simulink model "test_RS_flipflop_statemachine"  (R2021a)
settings: Solver=FixedStepDiscrete  StartTime=0.0  StopTime=210*10e-8  RelTol=1e-3
values from neighbouring files (symbols this model uses):
  t_ADC = 1/f_ADC    (= 1e-05)    [uz_6ph_pu_vsd_voltages_init.m]    (also in uz_mpc_6ph_init.m; uz_mpc_6ph_state_machine_init.m; uz_typeconv_init.m)
  t_clock = 1/f_clock    (= 1e-08)    [uz_6ph_pu_vsd_voltages_init.m]    (also in uz_mpc_6ph_init.m; uz_mpc_6ph_state_machine_init.m; uz_typeconv_init.m)
libraries: simulink x15, simulink_extras x1
settings Model: DataTypeOverride=Off  Creator=micha  LastModifiedBy=micha
settings SolverCC: AlgebraicLoopSolver=TrustRegion
settings DataIOCC: LimitDataPoints=on  SaveOutput=off  SaveTime=off
settings OptimizationCC: BlockReduction=off  ConditionallyExecuteInputs=off  DefaultParameterBehavior=Inlined  LifeSpan=inf
settings DebuggingCC: AlgebraicLoopMsg=error  SingleTaskRateTransMsg=error  AllowSymbolicDim=off  StrictBusMsg=ErrorOnBusTreatedAsVector  SFUnexpectedBacktrackingDiag=warning  SFNoUnconditionalDefaultTransitionDiag=warning  SFExecutionAtInitializationDiag=none  SFMachineParentedDataDiag=warning  ArithmeticOperatorsInVariantConditions=warning
settings HardwareCC: ProdBitPerPointer=32  ProdBitPerSizeT=32  ProdBitPerPtrDiffT=32  ProdLargestAtomicFloat=None  ProdIntDivRoundTo=Undefined  ProdEndianess=Unspecified  ProdWordSize=32  ProdHWDeviceType=ASIC/FPGA->ASIC/FPGA  ProdEqTarget=off
settings SFSimCC: SimUseLocalCustomCode=off  CustomCodeUndefinedFunction=UseInterfaceOnly
settings RTWCC: RTWUseLocalCustomCode=off
settings CodeAppCC: StateflowObjectComments=on
settings GRTTargetCC: TargetLangStandard=C89/C90 (ANSI)
settings ConfigComp: CovScope=ReferencedModels  CovMetricSettings=dw  CovSaveCumulativeToWorkspaceVar=on  CovSaveSingleToWorkspaceVar=on  CovExternalEMLEnable=off  CovSFcnEnable=off

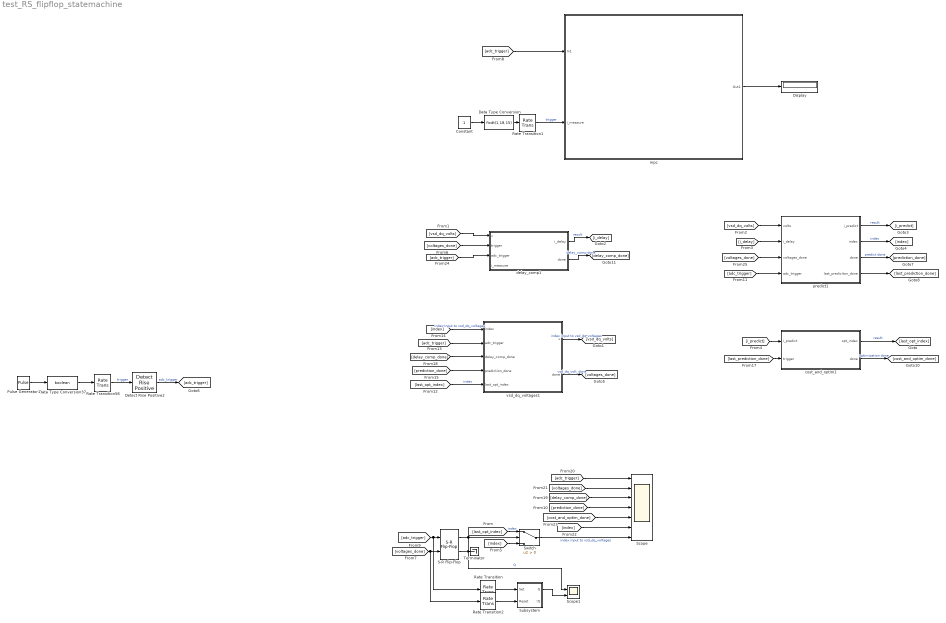
== system test_RS_flipflop_statemachine ==
  Constant : Constant
  Data Type Conversion : DataTypeConversion  OutDataTypeStr=fixdt(1,18,15)
  Data Type Conversion37 : DataTypeConversion  OutDataTypeStr=boolean
  Detect Rise Positive2 : simulink/Logic and Bit Operations/Detect Rise Positive  vinit=0  OutDataTypeStr=boolean
  Display : Display
  Pulse Generator1 : DiscretePulseGenerator  PulseType=Time based  Period=t_ADC  PulseWidth=5
  Rate Transition{,1..2,58} (4 alike) : RateTransition  OutPortSampleTime=t_clock
  S-R Flip-Flop : simulink_extras/Flip Flops/S-R Flip-Flop  initial_condition=0
  Scope : Scope  NumInputPorts=7
  Scope1 : Scope  NumInputPorts=2
  Subsystem : Subsystem
  Switch : Switch  Criteria=u2 > Threshold
  Terminator : Terminator
  cost_and_optim1 : Subsystem
  delay_comp1 : Subsystem
  mpc : Subsystem  TreatAsAtomicUnit=on
  predict1 : Subsystem
  vsd_dq_voltages1 : Subsystem
  wires:
  Data Type Conversion37/1 -> Rate Transition58/1
  Rate Transition58/1 -> Detect Rise Positive2/1  "trigger"
  Pulse Generator1/1 -> Data Type Conversion37/1
  S-R Flip-Flop/1 -> Scope1/1, Switch/2  "Q"
  [last_opt_index] -> Switch/1  "index"
  [index] -> vsd_dq_voltages1/1(index)  "index input to vsd_dq_voltages"
  S-R Flip-Flop/2 -> Terminator/1
  Detect Rise Positive2/1 -> [adc_trigger]  "adc_trigger"
  vsd_dq_voltages1/2(done) -> [voltages_done]  "vsd_dq_volt_done"
  predict1/3(done) -> [prediction_done]  "predict done"
  predict1/2(index) -> [index]  "index"
  cost_and_optim1/1(opt_index) -> [last_opt_index]  "result"
  [vsd_dq_volts] -> delay_comp1/1(v)
  [vsd_dq_volts] -> predict1/1(volts)
  delay_comp1/1(i_delay) -> [i_delay]  "result"
  [i_delay] -> predict1/2(i_delay)
  predict1/1(i_predict) -> [i_predict]  "result"
  [i_predict] -> cost_and_optim1/1(i_predict)
  [index] -> Switch/3
  [voltages_done] -> delay_comp1/2(trigger)
  [voltages_done] -> Rate Transition2/1, S-R Flip-Flop/2
  [adc_trigger] -> Rate Transition/1, S-R Flip-Flop/1
  [adc_trigger] -> predict1/4(adc_trigger)
  [last_opt_index] -> vsd_dq_voltages1/5(last_opt_index)  "index"
  [adc_trigger] -> vsd_dq_voltages1/2(adc_trigger)
  vsd_dq_voltages1/1(v) -> [vsd_dq_volts]  "index input to vsd_dq_voltages"
  [prediction_done] -> vsd_dq_voltages1/4(prediction_done)
  [last_prediction_done] -> cost_and_optim1/2(trigger)
  [delay_comp_done] -> vsd_dq_voltages1/3(delay_comp_done)
  Switch/1 -> Scope/7  "index input to vsd_dq_voltages"
  [delay_comp_done] -> Scope/3
  [adc_trigger] -> Scope/1
  [voltages_done] -> Scope/2
  [index] -> Scope/6
  cost_and_optim1/2(done) -> [cost_and_optim_done]  "optimization done"
  [cost_and_optim_done] -> Scope/5
  [adc_trigger] -> delay_comp1/3(adc_trigger)
  delay_comp1/2(done) -> [delay_comp_done]  "delay_comp done"
  [voltages_done] -> predict1/3(voltages_done)
  predict1/4(last_prediciton_done) -> [last_prediction_done]
  [prediction_done] -> Scope/4
  [adc_trigger] -> mpc/1(In1)
  Rate Transition1/1 -> mpc/2(i_measure)  "trigger"
  Constant/1 -> Data Type Conversion/1
  Data Type Conversion/1 -> Rate Transition1/1
  mpc/1(Out1) -> Display/1
  Subsystem/1(Q) -> Scope1/2
  Rate Transition/1 -> Subsystem/1(Set)
  Rate Transition2/1 -> Subsystem/2(Reset)

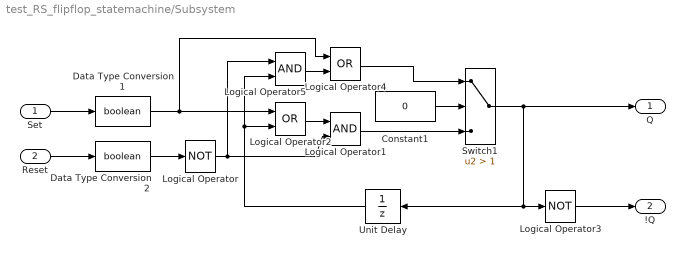
== system test_RS_flipflop_statemachine/Subsystem ==
  Set : Inport
  Reset : Inport  Port=2
  Constant1 : Constant  Value=0  SampleTime=-1
  Data Type Conversion1 : DataTypeConversion  OutDataTypeStr=boolean
  Data Type Conversion2 : DataTypeConversion  OutDataTypeStr=boolean
  Logical Operator : Logic  Operator=NOT  AllPortsSameDT=off  OutDataTypeStr=boolean
  Logical Operator1 : Logic  AllPortsSameDT=off  OutDataTypeStr=boolean
  Logical Operator2 : Logic  Operator=OR  AllPortsSameDT=off  OutDataTypeStr=boolean
  Logical Operator3 : Logic  Operator=NOT  AllPortsSameDT=off  OutDataTypeStr=boolean
  Logical Operator4 : Logic  Operator=OR  AllPortsSameDT=off  OutDataTypeStr=boolean
  Logical Operator5 : Logic  AllPortsSameDT=off  OutDataTypeStr=boolean
  Switch1 : Switch  Criteria=u2 > Threshold  Threshold=1
  Unit Delay : UnitDelay  SampleTime=t_clock  HasFrameUpgradeWarning=on
  Q : Outport  VectorParamsAs1DForOutWhenUnconnected=off
  !Q : Outport  Port=2  VectorParamsAs1DForOutWhenUnconnected=off
  wires:
  Logical Operator/1 -> Logical Operator1/2, Logical Operator5/1
  Reset/1 -> Data Type Conversion2/1
  Constant1/1 -> Switch1/2
  Logical Operator4/1 -> Switch1/1
  Data Type Conversion1/1 -> Logical Operator2/1, Logical Operator4/1
  Switch1/1 -> Q/1, Unit Delay/1, Logical Operator3/1
  Logical Operator3/1 -> !Q/1
  Set/1 -> Data Type Conversion1/1
  Logical Operator2/1 -> Logical Operator1/1
  Unit Delay/1 -> Logical Operator2/2, Logical Operator5/2
  Logical Operator5/1 -> Logical Operator4/2
  Logical Operator1/1 -> Switch1/3
  Data Type Conversion2/1 -> Logical Operator/1

== system test_RS_flipflop_statemachine/cost_and_optim1 ==
  i_predict : Inport
  trigger : Inport  Port=2
  Add : Sum
  Constant : Constant  Value=42  OutDataTypeStr=uint32  SampleTime=-1
  Delay{,1..4} (5 alike) : Delay  DelayLength=1
  Detect Rise Positive : simulink/Logic and Bit Operations/Detect Rise Positive  vinit=0  OutDataTypeStr=boolean
  Switch : Switch  Criteria=u2 > Threshold
  Terminator : Terminator
  opt_index : Outport  VectorParamsAs1DForOutWhenUnconnected=off
  done : Outport  Port=2  VectorParamsAs1DForOutWhenUnconnected=off
  wires:
  trigger/1 -> Delay/1
  Delay/1 -> Detect Rise Positive/1
  Delay1/1 -> done/1
  Detect Rise Positive/1 -> Delay1/1, Switch/2
  Delay2/1 -> Switch/3
  Switch/1 -> Add/1, Add/2, Delay2/1
  i_predict/1 -> Delay3/1
  Delay3/1 -> Switch/1
  Delay4/1 -> opt_index/1
  Constant/1 -> Delay4/1
  Add/1 -> Terminator/1

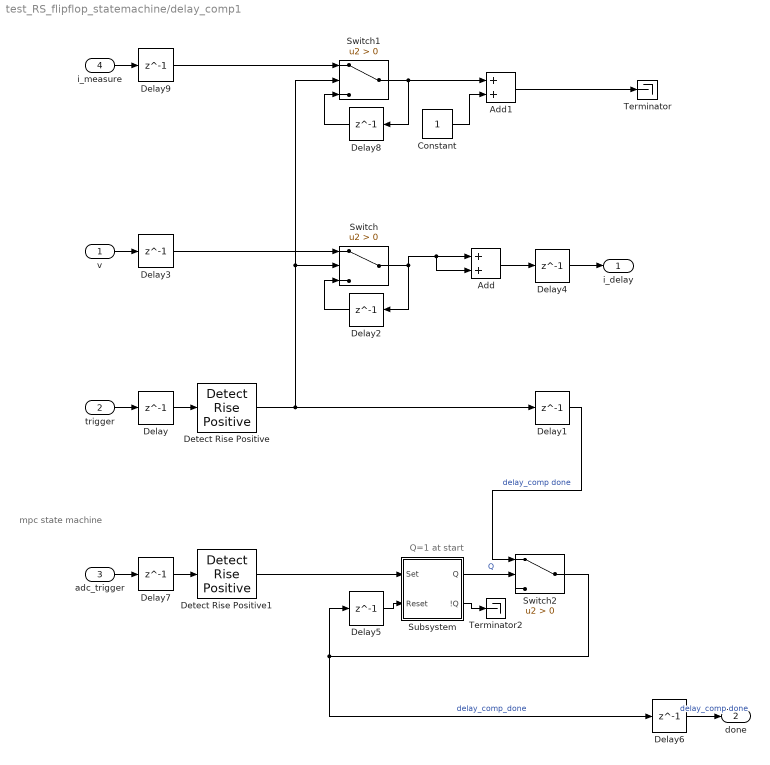
== system test_RS_flipflop_statemachine/delay_comp1 ==
  note: mpc state machine
  note: Q=1 at start
  v : Inport
  trigger : Inport  Port=2
  adc_trigger : Inport  Port=3
  i_measure : Inport  Port=4
  Add : Sum
  Add1 : Sum  AccumDataTypeStr=fixdt(1,18,15)
  Constant : Constant  OutDataTypeStr=fixdt(1,27,24)  SampleTime=-1
  Delay{,1..9} (10 alike) : Delay  DelayLength=1
  Detect Rise Positive : simulink/Logic and Bit Operations/Detect Rise Positive  vinit=0  OutDataTypeStr=boolean
  Detect Rise Positive1 : simulink/Logic and Bit Operations/Detect Rise Positive  vinit=0  OutDataTypeStr=boolean
  Subsystem : Subsystem
  Switch : Switch  Criteria=u2 > Threshold
  Switch1 : Switch  Criteria=u2 > Threshold
  Switch2 : Switch  Criteria=u2 > Threshold
  Terminator : Terminator
  Terminator2 : Terminator
  i_delay : Outport  VectorParamsAs1DForOutWhenUnconnected=off
  done : Outport  Port=2  VectorParamsAs1DForOutWhenUnconnected=off
  wires:
  trigger/1 -> Delay/1
  Delay/1 -> Detect Rise Positive/1
  Delay2/1 -> Switch/3
  Switch/1 -> Add/2, Add/1, Delay2/1
  v/1 -> Delay3/1
  Delay3/1 -> Switch/1
  Delay4/1 -> i_delay/1
  Add/1 -> Delay4/1
  Switch2/1 -> Delay5/1, Delay6/1  "delay_comp_done"
  Subsystem/1(Q) -> Switch2/2  "Q"
  Delay7/1 -> Detect Rise Positive1/1
  Subsystem/2(!Q) -> Terminator2/1
  Delay5/1 -> Subsystem/2(Reset)
  Delay1/1 -> Switch2/1  "delay_comp done"
  Delay6/1 -> done/1  "delay_comp done"
  adc_trigger/1 -> Delay7/1
  Detect Rise Positive1/1 -> Subsystem/1(Set)
  Detect Rise Positive/1 -> Delay1/1, Switch1/2, Switch/2
  i_measure/1 -> Delay9/1
  Switch1/1 -> Add1/1, Delay8/1
  Delay8/1 -> Switch1/3
  Delay9/1 -> Switch1/1
  Constant/1 -> Add1/2
  Add1/1 -> Terminator/1

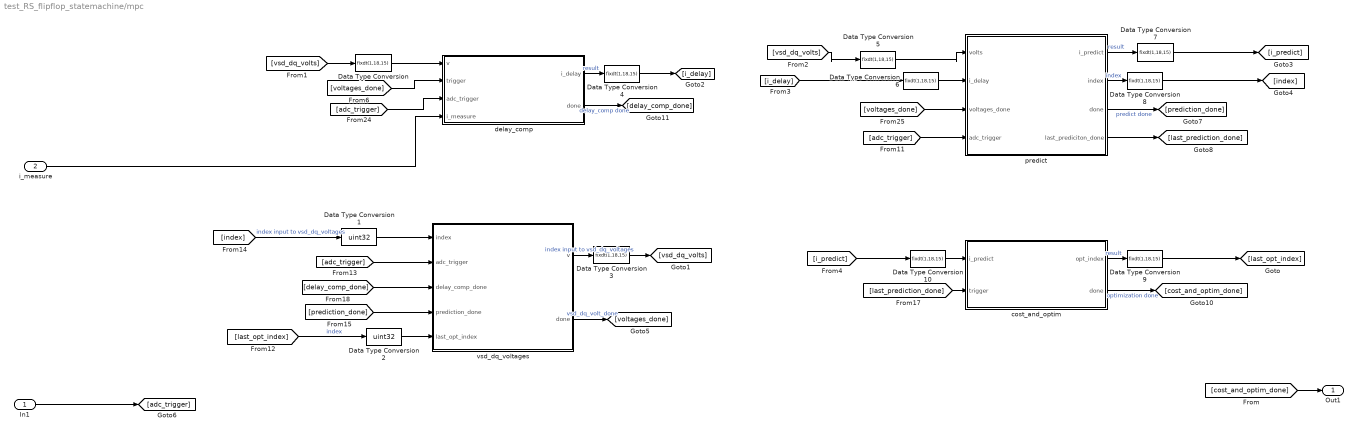
== system test_RS_flipflop_statemachine/mpc ==
  In1 : Inport
  i_measure : Inport  Port=2
  Data Type Conversion{,3..10} (9 alike) : DataTypeConversion  OutDataTypeStr=fixdt(1,18,15)
  Data Type Conversion1 : DataTypeConversion  OutDataTypeStr=uint32
  Data Type Conversion2 : DataTypeConversion  OutDataTypeStr=uint32
  cost_and_optim : Subsystem
  delay_comp : Subsystem
  predict : Subsystem
  vsd_dq_voltages : Subsystem
  Out1 : Outport
  wires:
  cost_and_optim/2(done) -> [cost_and_optim_done]  "optimization done"
  [voltages_done] -> predict/3(voltages_done)
  predict/4(last_prediciton_done) -> [last_prediction_done]
  [prediction_done] -> vsd_dq_voltages/4(prediction_done)
  delay_comp/2(done) -> [delay_comp_done]  "delay_comp done"
  [adc_trigger] -> vsd_dq_voltages/2(adc_trigger)
  [adc_trigger] -> predict/4(adc_trigger)
  [voltages_done] -> delay_comp/2(trigger)
  [vsd_dq_volts] -> Data Type Conversion/1
  [vsd_dq_volts] -> Data Type Conversion5/1
  [last_opt_index] -> Data Type Conversion2/1  "index"
  [i_delay] -> Data Type Conversion6/1
  delay_comp/1(i_delay) -> Data Type Conversion4/1  "result"
  cost_and_optim/1(opt_index) -> Data Type Conversion9/1  "result"
  vsd_dq_voltages/1(v) -> Data Type Conversion3/1  "index input to vsd_dq_voltages"
  [i_predict] -> Data Type Conversion10/1
  predict/1(i_predict) -> Data Type Conversion7/1  "result"
  [last_prediction_done] -> cost_and_optim/2(trigger)
  [index] -> Data Type Conversion1/1  "index input to vsd_dq_voltages"
  predict/3(done) -> [prediction_done]  "predict done"
  vsd_dq_voltages/2(done) -> [voltages_done]  "vsd_dq_volt_done"
  predict/2(index) -> Data Type Conversion8/1  "index"
  [delay_comp_done] -> vsd_dq_voltages/3(delay_comp_done)
  [adc_trigger] -> delay_comp/3(adc_trigger)
  In1/1 -> [adc_trigger]
  [cost_and_optim_done] -> Out1/1
  i_measure/1 -> delay_comp/4(i_measure)
  Data Type Conversion/1 -> delay_comp/1(v)
  Data Type Conversion1/1 -> vsd_dq_voltages/1(index)
  Data Type Conversion2/1 -> vsd_dq_voltages/5(last_opt_index)
  Data Type Conversion3/1 -> [vsd_dq_volts]
  Data Type Conversion4/1 -> [i_delay]
  Data Type Conversion5/1 -> predict/1(volts)
  Data Type Conversion6/1 -> predict/2(i_delay)
  Data Type Conversion7/1 -> [i_predict]
  Data Type Conversion8/1 -> [index]
  Data Type Conversion9/1 -> [last_opt_index]
  Data Type Conversion10/1 -> cost_and_optim/1(i_predict)

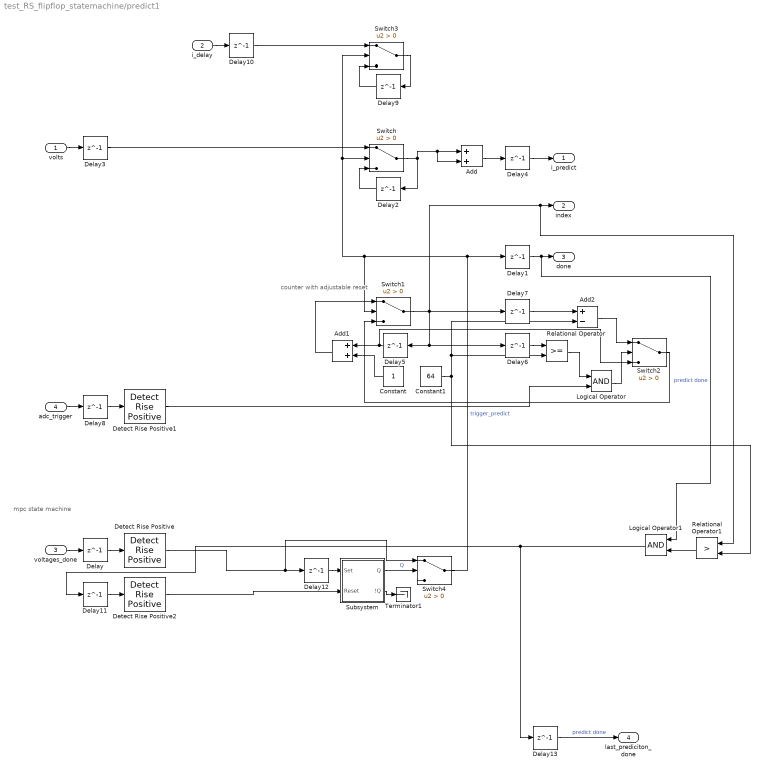
== system test_RS_flipflop_statemachine/predict1 ==
  note: counter with adjustable reset
  note: mpc state machine
  volts : Inport
  i_delay : Inport  Port=2
  voltages_done : Inport  Port=3
  adc_trigger : Inport  Port=4
  Add : Sum
  Add1 : Sum  AccumDataTypeStr=uint32
  Add2 : Sum  Inputs=+-  AccumDataTypeStr=uint32
  Constant : Constant  OutDataTypeStr=uint32  SampleTime=-1
  Constant1 : Constant  Value=64  OutDataTypeStr=uint32  SampleTime=-1
  Delay{,1..4,8..13} (11 alike) : Delay  DelayLength=1
  Delay5 : Delay  DelayLength=1  InitialCondition=1
  Delay6 : Delay  DelayLength=1  InitialCondition=1
  Delay7 : Delay  DelayLength=1  InitialCondition=1
  Detect Rise Positive : simulink/Logic and Bit Operations/Detect Rise Positive  vinit=0  OutDataTypeStr=boolean
  Detect Rise Positive1 : simulink/Logic and Bit Operations/Detect Rise Positive  vinit=0  OutDataTypeStr=boolean
  Detect Rise Positive2 : simulink/Logic and Bit Operations/Detect Rise Positive  vinit=0  OutDataTypeStr=boolean
  Logical Operator : Logic  AllPortsSameDT=off  OutDataTypeStr=boolean
  Logical Operator1 : Logic  AllPortsSameDT=off  OutDataTypeStr=boolean
  Relational Operator : RelationalOperator  OutDataTypeStr=boolean  RndMeth=Simplest
  Relational Operator1 : RelationalOperator  Operator=>  OutDataTypeStr=boolean  RndMeth=Simplest
  Subsystem : Subsystem
  Switch{,1..4} (5 alike) : Switch  Criteria=u2 > Threshold
  Terminator1 : Terminator
  i_predict : Outport  VectorParamsAs1DForOutWhenUnconnected=off
  index : Outport  Port=2  VectorParamsAs1DForOutWhenUnconnected=off
  done : Outport  Port=3  VectorParamsAs1DForOutWhenUnconnected=off
  last_prediciton_done : Outport  Port=4  VectorParamsAs1DForOutWhenUnconnected=off
  wires:
  voltages_done/1 -> Delay/1
  Delay/1 -> Detect Rise Positive/1
  Delay2/1 -> Switch/3
  Switch/1 -> Add/2, Add/1, Delay2/1
  volts/1 -> Delay3/1
  Delay3/1 -> Switch/1
  Delay4/1 -> i_predict/1
  Add/1 -> Delay4/1
  Delay5/1 -> Switch2/3, Add1/1
  Constant/1 -> Add1/2
  Add1/1 -> Switch1/1
  Constant1/1 -> Relational Operator1/2, Add2/2, Relational Operator/2
  Relational Operator/1 -> Logical Operator/1
  Switch2/1 -> Switch1/3
  Add2/1 -> Switch2/1
  Delay6/1 -> Relational Operator/1
  Delay7/1 -> Add2/1
  Logical Operator/1 -> Switch2/2
  Delay8/1 -> Detect Rise Positive1/1
  adc_trigger/1 -> Delay8/1
  Detect Rise Positive1/1 -> Logical Operator/2
  i_delay/1 -> Delay10/1
  Delay9/1 -> Switch3/3
  Delay10/1 -> Switch3/1
  Switch3/1 -> Delay9/1
  Delay11/1 -> Detect Rise Positive2/1
  Logical Operator1/1 -> Delay13/1, Delay11/1
  Switch4/1 -> Delay1/1, Switch3/2, Switch/2, Switch1/2  "trigger_predict"
  Detect Rise Positive2/1 -> Subsystem/2(Reset)
  Detect Rise Positive/1 -> Switch4/1, Delay12/1
  Delay12/1 -> Subsystem/1(Set)
  Subsystem/2(!Q) -> Terminator1/1
  Subsystem/1(Q) -> Switch4/2  "Q"
  Relational Operator1/1 -> Logical Operator1/2
  Switch1/1 -> Delay5/1, Delay6/1, Delay7/1, Relational Operator1/1, index/1
  Delay1/1 -> Logical Operator1/1, done/1  "predict done"
  Delay13/1 -> last_prediciton_done/1  "predict done"

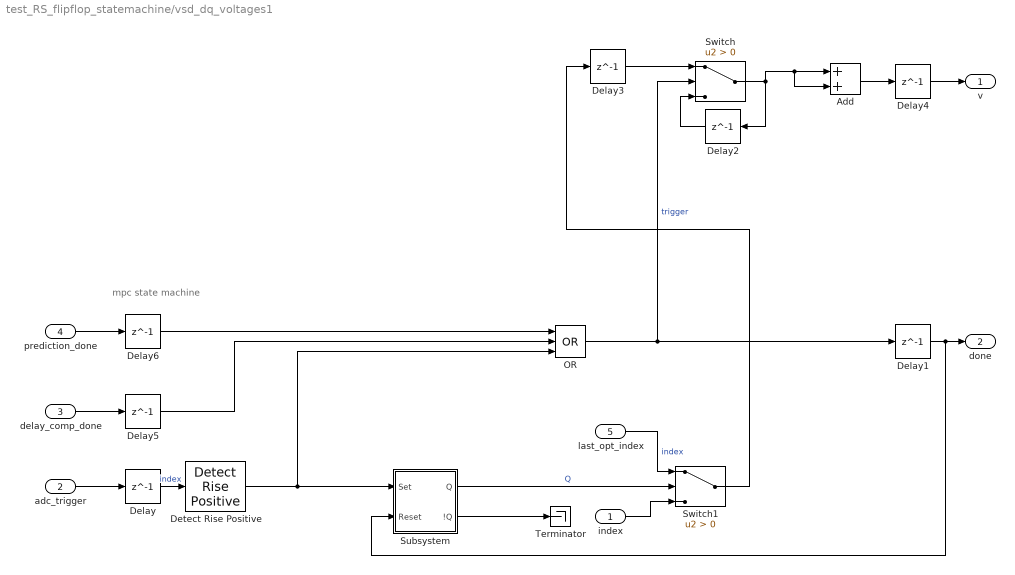
== system test_RS_flipflop_statemachine/vsd_dq_voltages1 ==
  note: mpc state machine
  index : Inport
  adc_trigger : Inport  Port=2
  delay_comp_done : Inport  Port=3
  prediction_done : Inport  Port=4
  last_opt_index : Inport  Port=5
  Add : Sum
  Delay{,1..6} (7 alike) : Delay  DelayLength=1
  Detect Rise Positive : simulink/Logic and Bit Operations/Detect Rise Positive  vinit=0  OutDataTypeStr=boolean
  OR : Logic  Operator=OR  Inputs=3  IconShape=distinctive  AllPortsSameDT=off  OutDataTypeStr=boolean
  Subsystem : Subsystem
  Switch : Switch  Criteria=u2 > Threshold
  Switch1 : Switch  Criteria=u2 > Threshold
  Terminator : Terminator
  v : Outport  VectorParamsAs1DForOutWhenUnconnected=off
  done : Outport  Port=2  VectorParamsAs1DForOutWhenUnconnected=off
  wires:
  Delay1/1 -> Subsystem/2(Reset), done/1
  Delay2/1 -> Switch/3
  Switch/1 -> Add/2, Add/1, Delay2/1
  Switch1/1 -> Delay3/1
  Delay3/1 -> Switch/1
  Delay4/1 -> v/1
  Add/1 -> Delay4/1
  adc_trigger/1 -> Delay/1
  Detect Rise Positive/1 -> OR/3, Subsystem/1(Set)
  OR/1 -> Switch/2, Delay1/1  "trigger"
  delay_comp_done/1 -> Delay5/1
  prediction_done/1 -> Delay6/1
  Delay5/1 -> OR/2
  Delay6/1 -> OR/1
  Subsystem/2(!Q) -> Terminator/1
  index/1 -> Switch1/3
  Subsystem/1(Q) -> Switch1/2  "Q"
  last_opt_index/1 -> Switch1/1  "index"
  Delay/1 -> Detect Rise Positive/1  "index"

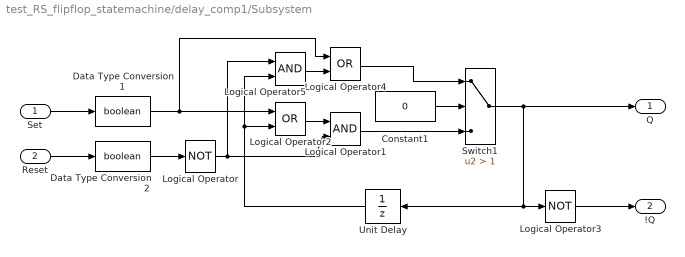
== system test_RS_flipflop_statemachine/delay_comp1/Subsystem ==
  Set : Inport
  Reset : Inport  Port=2
  Constant1 : Constant  Value=0  OutDataTypeStr=uint32  SampleTime=-1
  Data Type Conversion1 : DataTypeConversion  OutDataTypeStr=boolean
  Data Type Conversion2 : DataTypeConversion  OutDataTypeStr=boolean
  Logical Operator : Logic  Operator=NOT  AllPortsSameDT=off  OutDataTypeStr=boolean
  Logical Operator1 : Logic  AllPortsSameDT=off  OutDataTypeStr=boolean
  Logical Operator2 : Logic  Operator=OR  AllPortsSameDT=off  OutDataTypeStr=boolean
  Logical Operator3 : Logic  Operator=NOT  AllPortsSameDT=off  OutDataTypeStr=boolean
  Logical Operator4 : Logic  Operator=OR  AllPortsSameDT=off  OutDataTypeStr=boolean
  Logical Operator5 : Logic  AllPortsSameDT=off  OutDataTypeStr=boolean
  Switch1 : Switch  Criteria=u2 > Threshold  Threshold=1
  Unit Delay : UnitDelay  InitialCondition=1  SampleTime=t_clock  HasFrameUpgradeWarning=on
  Q : Outport  VectorParamsAs1DForOutWhenUnconnected=off
  !Q : Outport  Port=2  VectorParamsAs1DForOutWhenUnconnected=off
  wires:
  Logical Operator/1 -> Logical Operator1/2, Logical Operator5/1
  Reset/1 -> Data Type Conversion2/1
  Constant1/1 -> Switch1/2
  Logical Operator4/1 -> Switch1/1
  Data Type Conversion1/1 -> Logical Operator2/1, Logical Operator4/1
  Switch1/1 -> Q/1, Unit Delay/1, Logical Operator3/1
  Logical Operator3/1 -> !Q/1
  Set/1 -> Data Type Conversion1/1
  Logical Operator2/1 -> Logical Operator1/1
  Unit Delay/1 -> Logical Operator2/2, Logical Operator5/2
  Logical Operator5/1 -> Logical Operator4/2
  Logical Operator1/1 -> Switch1/3
  Data Type Conversion2/1 -> Logical Operator/1

== system test_RS_flipflop_statemachine/mpc/cost_and_optim ==
  i_predict : Inport
  trigger : Inport  Port=2
  Add : Sum
  Constant : Constant  Value=42  OutDataTypeStr=uint32  SampleTime=-1
  Delay{,1..4} (5 alike) : Delay  DelayLength=1
  Detect Rise Positive : simulink/Logic and Bit Operations/Detect Rise Positive  vinit=0  OutDataTypeStr=boolean
  Switch : Switch  Criteria=u2 > Threshold
  Terminator : Terminator
  opt_index : Outport  VectorParamsAs1DForOutWhenUnconnected=off
  done : Outport  Port=2  VectorParamsAs1DForOutWhenUnconnected=off
  wires:
  trigger/1 -> Delay/1
  Delay/1 -> Detect Rise Positive/1
  Delay1/1 -> done/1
  Detect Rise Positive/1 -> Delay1/1, Switch/2
  Delay2/1 -> Switch/3
  Switch/1 -> Add/1, Add/2, Delay2/1
  i_predict/1 -> Delay3/1
  Delay3/1 -> Switch/1
  Delay4/1 -> opt_index/1
  Constant/1 -> Delay4/1
  Add/1 -> Terminator/1

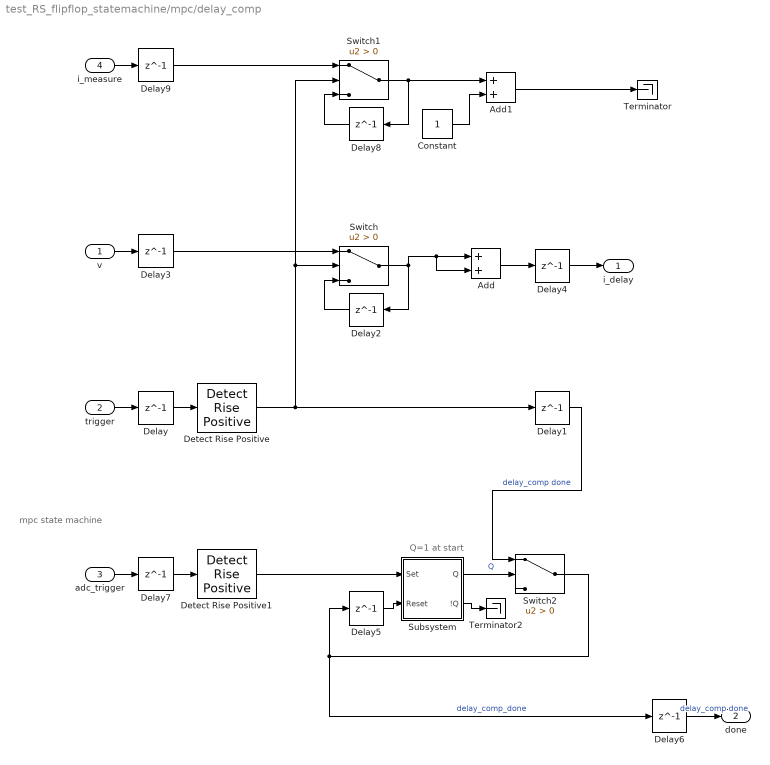
== system test_RS_flipflop_statemachine/mpc/delay_comp ==
  note: mpc state machine
  note: Q=1 at start
  v : Inport
  trigger : Inport  Port=2
  adc_trigger : Inport  Port=3
  i_measure : Inport  Port=4
  Add : Sum
  Add1 : Sum  AccumDataTypeStr=fixdt(1,18,15)
  Constant : Constant  OutDataTypeStr=fixdt(1,27,24)  SampleTime=-1
  Delay{,1..9} (10 alike) : Delay  DelayLength=1
  Detect Rise Positive : simulink/Logic and Bit Operations/Detect Rise Positive  vinit=0  OutDataTypeStr=boolean
  Detect Rise Positive1 : simulink/Logic and Bit Operations/Detect Rise Positive  vinit=0  OutDataTypeStr=boolean
  Subsystem : Subsystem
  Switch : Switch  Criteria=u2 > Threshold
  Switch1 : Switch  Criteria=u2 > Threshold
  Switch2 : Switch  Criteria=u2 > Threshold
  Terminator : Terminator
  Terminator2 : Terminator
  i_delay : Outport  VectorParamsAs1DForOutWhenUnconnected=off
  done : Outport  Port=2  VectorParamsAs1DForOutWhenUnconnected=off
  wires:
  trigger/1 -> Delay/1
  Delay/1 -> Detect Rise Positive/1
  Delay2/1 -> Switch/3
  Switch/1 -> Add/2, Add/1, Delay2/1
  v/1 -> Delay3/1
  Delay3/1 -> Switch/1
  Delay4/1 -> i_delay/1
  Add/1 -> Delay4/1
  Switch2/1 -> Delay5/1, Delay6/1  "delay_comp_done"
  Subsystem/1(Q) -> Switch2/2  "Q"
  Delay7/1 -> Detect Rise Positive1/1
  Subsystem/2(!Q) -> Terminator2/1
  Delay5/1 -> Subsystem/2(Reset)
  Delay1/1 -> Switch2/1  "delay_comp done"
  Delay6/1 -> done/1  "delay_comp done"
  adc_trigger/1 -> Delay7/1
  Detect Rise Positive1/1 -> Subsystem/1(Set)
  Detect Rise Positive/1 -> Delay1/1, Switch1/2, Switch/2
  i_measure/1 -> Delay9/1
  Switch1/1 -> Add1/1, Delay8/1
  Delay8/1 -> Switch1/3
  Delay9/1 -> Switch1/1
  Constant/1 -> Add1/2
  Add1/1 -> Terminator/1

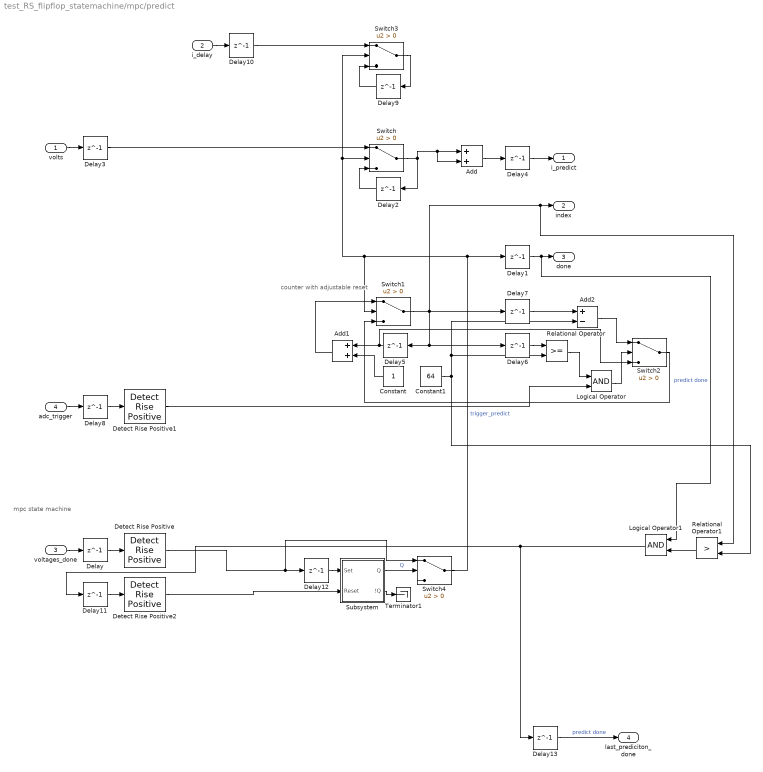
== system test_RS_flipflop_statemachine/mpc/predict ==
  note: counter with adjustable reset
  note: mpc state machine
  volts : Inport
  i_delay : Inport  Port=2
  voltages_done : Inport  Port=3
  adc_trigger : Inport  Port=4
  Add : Sum
  Add1 : Sum  AccumDataTypeStr=uint32
  Add2 : Sum  Inputs=+-  AccumDataTypeStr=uint32
  Constant : Constant  OutDataTypeStr=uint32  SampleTime=-1
  Constant1 : Constant  Value=64  OutDataTypeStr=uint32  SampleTime=-1
  Delay{,1..4,8..13} (11 alike) : Delay  DelayLength=1
  Delay5 : Delay  DelayLength=1  InitialCondition=1
  Delay6 : Delay  DelayLength=1  InitialCondition=1
  Delay7 : Delay  DelayLength=1  InitialCondition=1
  Detect Rise Positive : simulink/Logic and Bit Operations/Detect Rise Positive  vinit=0  OutDataTypeStr=boolean
  Detect Rise Positive1 : simulink/Logic and Bit Operations/Detect Rise Positive  vinit=0  OutDataTypeStr=boolean
  Detect Rise Positive2 : simulink/Logic and Bit Operations/Detect Rise Positive  vinit=0  OutDataTypeStr=boolean
  Logical Operator : Logic  AllPortsSameDT=off  OutDataTypeStr=boolean
  Logical Operator1 : Logic  AllPortsSameDT=off  OutDataTypeStr=boolean
  Relational Operator : RelationalOperator  OutDataTypeStr=boolean  RndMeth=Simplest
  Relational Operator1 : RelationalOperator  Operator=>  OutDataTypeStr=boolean  RndMeth=Simplest
  Subsystem : Subsystem
  Switch{,1..4} (5 alike) : Switch  Criteria=u2 > Threshold
  Terminator1 : Terminator
  i_predict : Outport  VectorParamsAs1DForOutWhenUnconnected=off
  index : Outport  Port=2  VectorParamsAs1DForOutWhenUnconnected=off
  done : Outport  Port=3  VectorParamsAs1DForOutWhenUnconnected=off
  last_prediciton_done : Outport  Port=4  VectorParamsAs1DForOutWhenUnconnected=off
  wires:
  voltages_done/1 -> Delay/1
  Delay/1 -> Detect Rise Positive/1
  Delay2/1 -> Switch/3
  Switch/1 -> Add/2, Add/1, Delay2/1
  volts/1 -> Delay3/1
  Delay3/1 -> Switch/1
  Delay4/1 -> i_predict/1
  Add/1 -> Delay4/1
  Delay5/1 -> Switch2/3, Add1/1
  Constant/1 -> Add1/2
  Add1/1 -> Switch1/1
  Constant1/1 -> Relational Operator1/2, Add2/2, Relational Operator/2
  Relational Operator/1 -> Logical Operator/1
  Switch2/1 -> Switch1/3
  Add2/1 -> Switch2/1
  Delay6/1 -> Relational Operator/1
  Delay7/1 -> Add2/1
  Logical Operator/1 -> Switch2/2
  Delay8/1 -> Detect Rise Positive1/1
  adc_trigger/1 -> Delay8/1
  Detect Rise Positive1/1 -> Logical Operator/2
  i_delay/1 -> Delay10/1
  Delay9/1 -> Switch3/3
  Delay10/1 -> Switch3/1
  Switch3/1 -> Delay9/1
  Delay11/1 -> Detect Rise Positive2/1
  Logical Operator1/1 -> Delay13/1, Delay11/1
  Switch4/1 -> Delay1/1, Switch3/2, Switch/2, Switch1/2  "trigger_predict"
  Detect Rise Positive2/1 -> Subsystem/2(Reset)
  Detect Rise Positive/1 -> Switch4/1, Delay12/1
  Delay12/1 -> Subsystem/1(Set)
  Subsystem/2(!Q) -> Terminator1/1
  Subsystem/1(Q) -> Switch4/2  "Q"
  Relational Operator1/1 -> Logical Operator1/2
  Switch1/1 -> Delay5/1, Delay6/1, Delay7/1, Relational Operator1/1, index/1
  Delay1/1 -> Logical Operator1/1, done/1  "predict done"
  Delay13/1 -> last_prediciton_done/1  "predict done"

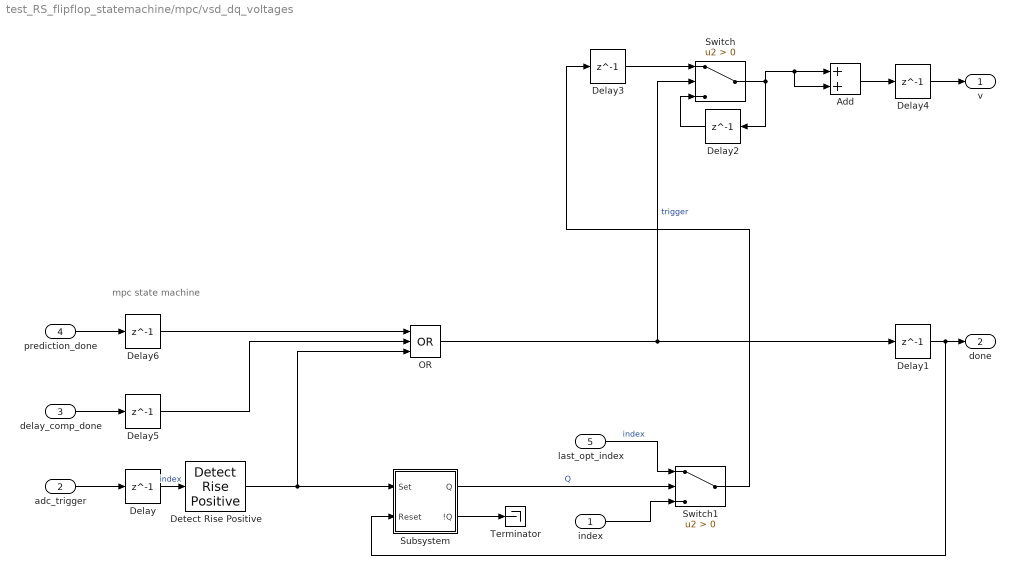
== system test_RS_flipflop_statemachine/mpc/vsd_dq_voltages ==
  note: mpc state machine
  index : Inport
  adc_trigger : Inport  Port=2
  delay_comp_done : Inport  Port=3
  prediction_done : Inport  Port=4
  last_opt_index : Inport  Port=5
  Add : Sum
  Delay{,1..6} (7 alike) : Delay  DelayLength=1
  Detect Rise Positive : simulink/Logic and Bit Operations/Detect Rise Positive  vinit=0  OutDataTypeStr=boolean
  OR : Logic  Operator=OR  Inputs=3  IconShape=distinctive  AllPortsSameDT=off  OutDataTypeStr=boolean
  Subsystem : Subsystem
  Switch : Switch  Criteria=u2 > Threshold
  Switch1 : Switch  Criteria=u2 > Threshold
  Terminator : Terminator
  v : Outport  VectorParamsAs1DForOutWhenUnconnected=off
  done : Outport  Port=2  VectorParamsAs1DForOutWhenUnconnected=off
  wires:
  Delay1/1 -> Subsystem/2(Reset), done/1
  Delay2/1 -> Switch/3
  Switch/1 -> Add/2, Add/1, Delay2/1
  Switch1/1 -> Delay3/1
  Delay3/1 -> Switch/1
  Delay4/1 -> v/1
  Add/1 -> Delay4/1
  adc_trigger/1 -> Delay/1
  Detect Rise Positive/1 -> OR/3, Subsystem/1(Set)
  OR/1 -> Switch/2, Delay1/1  "trigger"
  delay_comp_done/1 -> Delay5/1
  prediction_done/1 -> Delay6/1
  Delay5/1 -> OR/2
  Delay6/1 -> OR/1
  Subsystem/2(!Q) -> Terminator/1
  index/1 -> Switch1/3
  Subsystem/1(Q) -> Switch1/2  "Q"
  last_opt_index/1 -> Switch1/1  "index"
  Delay/1 -> Detect Rise Positive/1  "index"

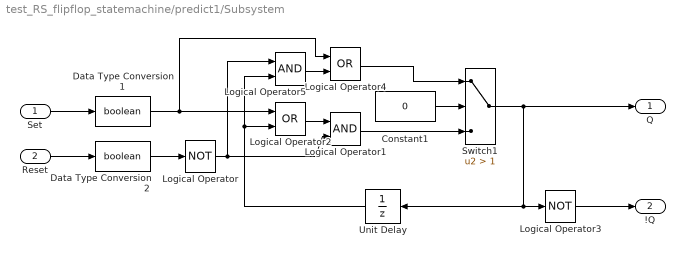
== system test_RS_flipflop_statemachine/predict1/Subsystem ==
  Set : Inport
  Reset : Inport  Port=2
  Constant1 : Constant  Value=0  OutDataTypeStr=uint32  SampleTime=-1
  Data Type Conversion1 : DataTypeConversion  OutDataTypeStr=boolean
  Data Type Conversion2 : DataTypeConversion  OutDataTypeStr=boolean
  Logical Operator : Logic  Operator=NOT  AllPortsSameDT=off  OutDataTypeStr=boolean
  Logical Operator1 : Logic  AllPortsSameDT=off  OutDataTypeStr=boolean
  Logical Operator2 : Logic  Operator=OR  AllPortsSameDT=off  OutDataTypeStr=boolean
  Logical Operator3 : Logic  Operator=NOT  AllPortsSameDT=off  OutDataTypeStr=boolean
  Logical Operator4 : Logic  Operator=OR  AllPortsSameDT=off  OutDataTypeStr=boolean
  Logical Operator5 : Logic  AllPortsSameDT=off  OutDataTypeStr=boolean
  Switch1 : Switch  Criteria=u2 > Threshold  Threshold=1
  Unit Delay : UnitDelay  SampleTime=t_clock  HasFrameUpgradeWarning=on
  Q : Outport  VectorParamsAs1DForOutWhenUnconnected=off
  !Q : Outport  Port=2  VectorParamsAs1DForOutWhenUnconnected=off
  wires:
  Logical Operator/1 -> Logical Operator1/2, Logical Operator5/1
  Reset/1 -> Data Type Conversion2/1
  Constant1/1 -> Switch1/2
  Logical Operator4/1 -> Switch1/1
  Data Type Conversion1/1 -> Logical Operator2/1, Logical Operator4/1
  Switch1/1 -> Q/1, Unit Delay/1, Logical Operator3/1
  Logical Operator3/1 -> !Q/1
  Set/1 -> Data Type Conversion1/1
  Logical Operator2/1 -> Logical Operator1/1
  Unit Delay/1 -> Logical Operator2/2, Logical Operator5/2
  Logical Operator5/1 -> Logical Operator4/2
  Logical Operator1/1 -> Switch1/3
  Data Type Conversion2/1 -> Logical Operator/1

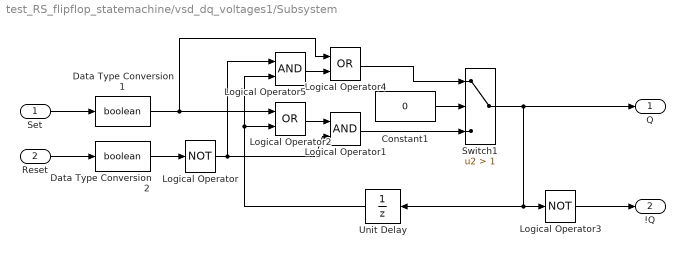
== system test_RS_flipflop_statemachine/vsd_dq_voltages1/Subsystem ==
  Set : Inport
  Reset : Inport  Port=2
  Constant1 : Constant  Value=0  OutDataTypeStr=uint32  SampleTime=-1
  Data Type Conversion1 : DataTypeConversion  OutDataTypeStr=boolean
  Data Type Conversion2 : DataTypeConversion  OutDataTypeStr=boolean
  Logical Operator : Logic  Operator=NOT  AllPortsSameDT=off  OutDataTypeStr=boolean
  Logical Operator1 : Logic  AllPortsSameDT=off  OutDataTypeStr=boolean
  Logical Operator2 : Logic  Operator=OR  AllPortsSameDT=off  OutDataTypeStr=boolean
  Logical Operator3 : Logic  Operator=NOT  AllPortsSameDT=off  OutDataTypeStr=boolean
  Logical Operator4 : Logic  Operator=OR  AllPortsSameDT=off  OutDataTypeStr=boolean
  Logical Operator5 : Logic  AllPortsSameDT=off  OutDataTypeStr=boolean
  Switch1 : Switch  Criteria=u2 > Threshold  Threshold=1
  Unit Delay : UnitDelay  SampleTime=t_clock  HasFrameUpgradeWarning=on
  Q : Outport  VectorParamsAs1DForOutWhenUnconnected=off
  !Q : Outport  Port=2  VectorParamsAs1DForOutWhenUnconnected=off
  wires:
  Logical Operator/1 -> Logical Operator1/2, Logical Operator5/1
  Reset/1 -> Data Type Conversion2/1
  Constant1/1 -> Switch1/2
  Logical Operator4/1 -> Switch1/1
  Data Type Conversion1/1 -> Logical Operator2/1, Logical Operator4/1
  Switch1/1 -> Q/1, Unit Delay/1, Logical Operator3/1
  Logical Operator3/1 -> !Q/1
  Set/1 -> Data Type Conversion1/1
  Logical Operator2/1 -> Logical Operator1/1
  Unit Delay/1 -> Logical Operator2/2, Logical Operator5/2
  Logical Operator5/1 -> Logical Operator4/2
  Logical Operator1/1 -> Switch1/3
  Data Type Conversion2/1 -> Logical Operator/1

== system test_RS_flipflop_statemachine/mpc/delay_comp/Subsystem ==
  Set : Inport
  Reset : Inport  Port=2
  Constant1 : Constant  Value=0  OutDataTypeStr=uint32  SampleTime=-1
  Data Type Conversion1 : DataTypeConversion  OutDataTypeStr=boolean
  Data Type Conversion2 : DataTypeConversion  OutDataTypeStr=boolean
  Logical Operator : Logic  Operator=NOT  AllPortsSameDT=off  OutDataTypeStr=boolean
  Logical Operator1 : Logic  AllPortsSameDT=off  OutDataTypeStr=boolean
  Logical Operator2 : Logic  Operator=OR  AllPortsSameDT=off  OutDataTypeStr=boolean
  Logical Operator3 : Logic  Operator=NOT  AllPortsSameDT=off  OutDataTypeStr=boolean
  Logical Operator4 : Logic  Operator=OR  AllPortsSameDT=off  OutDataTypeStr=boolean
  Logical Operator5 : Logic  AllPortsSameDT=off  OutDataTypeStr=boolean
  Switch1 : Switch  Criteria=u2 > Threshold  Threshold=1
  Unit Delay : UnitDelay  InitialCondition=1  SampleTime=t_clock  HasFrameUpgradeWarning=on
  Q : Outport  VectorParamsAs1DForOutWhenUnconnected=off
  !Q : Outport  Port=2  VectorParamsAs1DForOutWhenUnconnected=off
  wires:
  Logical Operator/1 -> Logical Operator1/2, Logical Operator5/1
  Reset/1 -> Data Type Conversion2/1
  Constant1/1 -> Switch1/2
  Logical Operator4/1 -> Switch1/1
  Data Type Conversion1/1 -> Logical Operator2/1, Logical Operator4/1
  Switch1/1 -> Q/1, Unit Delay/1, Logical Operator3/1
  Logical Operator3/1 -> !Q/1
  Set/1 -> Data Type Conversion1/1
  Logical Operator2/1 -> Logical Operator1/1
  Unit Delay/1 -> Logical Operator2/2, Logical Operator5/2
  Logical Operator5/1 -> Logical Operator4/2
  Logical Operator1/1 -> Switch1/3
  Data Type Conversion2/1 -> Logical Operator/1

== system test_RS_flipflop_statemachine/mpc/predict/Subsystem ==
  Set : Inport
  Reset : Inport  Port=2
  Constant1 : Constant  Value=0  OutDataTypeStr=uint32  SampleTime=-1
  Data Type Conversion1 : DataTypeConversion  OutDataTypeStr=boolean
  Data Type Conversion2 : DataTypeConversion  OutDataTypeStr=boolean
  Logical Operator : Logic  Operator=NOT  AllPortsSameDT=off  OutDataTypeStr=boolean
  Logical Operator1 : Logic  AllPortsSameDT=off  OutDataTypeStr=boolean
  Logical Operator2 : Logic  Operator=OR  AllPortsSameDT=off  OutDataTypeStr=boolean
  Logical Operator3 : Logic  Operator=NOT  AllPortsSameDT=off  OutDataTypeStr=boolean
  Logical Operator4 : Logic  Operator=OR  AllPortsSameDT=off  OutDataTypeStr=boolean
  Logical Operator5 : Logic  AllPortsSameDT=off  OutDataTypeStr=boolean
  Switch1 : Switch  Criteria=u2 > Threshold  Threshold=1
  Unit Delay : UnitDelay  SampleTime=t_clock  HasFrameUpgradeWarning=on
  Q : Outport  VectorParamsAs1DForOutWhenUnconnected=off
  !Q : Outport  Port=2  VectorParamsAs1DForOutWhenUnconnected=off
  wires:
  Logical Operator/1 -> Logical Operator1/2, Logical Operator5/1
  Reset/1 -> Data Type Conversion2/1
  Constant1/1 -> Switch1/2
  Logical Operator4/1 -> Switch1/1
  Data Type Conversion1/1 -> Logical Operator2/1, Logical Operator4/1
  Switch1/1 -> Q/1, Unit Delay/1, Logical Operator3/1
  Logical Operator3/1 -> !Q/1
  Set/1 -> Data Type Conversion1/1
  Logical Operator2/1 -> Logical Operator1/1
  Unit Delay/1 -> Logical Operator2/2, Logical Operator5/2
  Logical Operator5/1 -> Logical Operator4/2
  Logical Operator1/1 -> Switch1/3
  Data Type Conversion2/1 -> Logical Operator/1

== system test_RS_flipflop_statemachine/mpc/vsd_dq_voltages/Subsystem ==
  Set : Inport
  Reset : Inport  Port=2
  Constant1 : Constant  Value=0  OutDataTypeStr=uint32  SampleTime=-1
  Data Type Conversion1 : DataTypeConversion  OutDataTypeStr=boolean
  Data Type Conversion2 : DataTypeConversion  OutDataTypeStr=boolean
  Logical Operator : Logic  Operator=NOT  AllPortsSameDT=off  OutDataTypeStr=boolean
  Logical Operator1 : Logic  AllPortsSameDT=off  OutDataTypeStr=boolean
  Logical Operator2 : Logic  Operator=OR  AllPortsSameDT=off  OutDataTypeStr=boolean
  Logical Operator3 : Logic  Operator=NOT  AllPortsSameDT=off  OutDataTypeStr=boolean
  Logical Operator4 : Logic  Operator=OR  AllPortsSameDT=off  OutDataTypeStr=boolean
  Logical Operator5 : Logic  AllPortsSameDT=off  OutDataTypeStr=boolean
  Switch1 : Switch  Criteria=u2 > Threshold  Threshold=1
  Unit Delay : UnitDelay  SampleTime=t_clock  HasFrameUpgradeWarning=on
  Q : Outport  VectorParamsAs1DForOutWhenUnconnected=off
  !Q : Outport  Port=2  VectorParamsAs1DForOutWhenUnconnected=off
  wires:
  Logical Operator/1 -> Logical Operator1/2, Logical Operator5/1
  Reset/1 -> Data Type Conversion2/1
  Constant1/1 -> Switch1/2
  Logical Operator4/1 -> Switch1/1
  Data Type Conversion1/1 -> Logical Operator2/1, Logical Operator4/1
  Switch1/1 -> Q/1, Unit Delay/1, Logical Operator3/1
  Logical Operator3/1 -> !Q/1
  Set/1 -> Data Type Conversion1/1
  Logical Operator2/1 -> Logical Operator1/1
  Unit Delay/1 -> Logical Operator2/2, Logical Operator5/2
  Logical Operator5/1 -> Logical Operator4/2
  Logical Operator1/1 -> Switch1/3
  Data Type Conversion2/1 -> Logical Operator/1
